simulink model "ship_surface"  (R2026a)
settings: configuration reference "standardSILConfiguraitonParams" (kept outside this file)
undefined symbols (not defined in the file): vehicleParams
settings Model: Creator=jerem  LastModifiedBy=Edison Altamirano
settings ConfigSetRef: SourceName=standardSILConfiguraitonParams  SourceLocation=Base Workspace

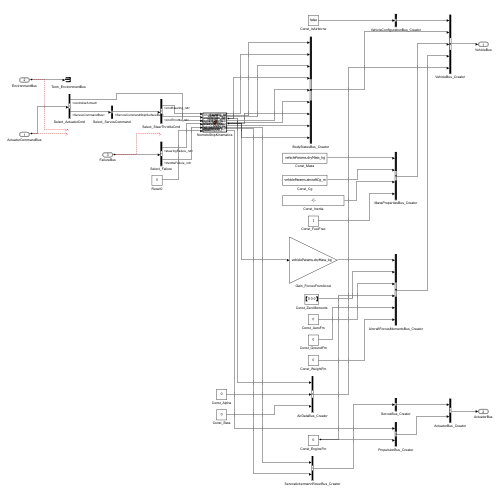
[thumbnail: Simulink's stored preview of the top-level diagram]
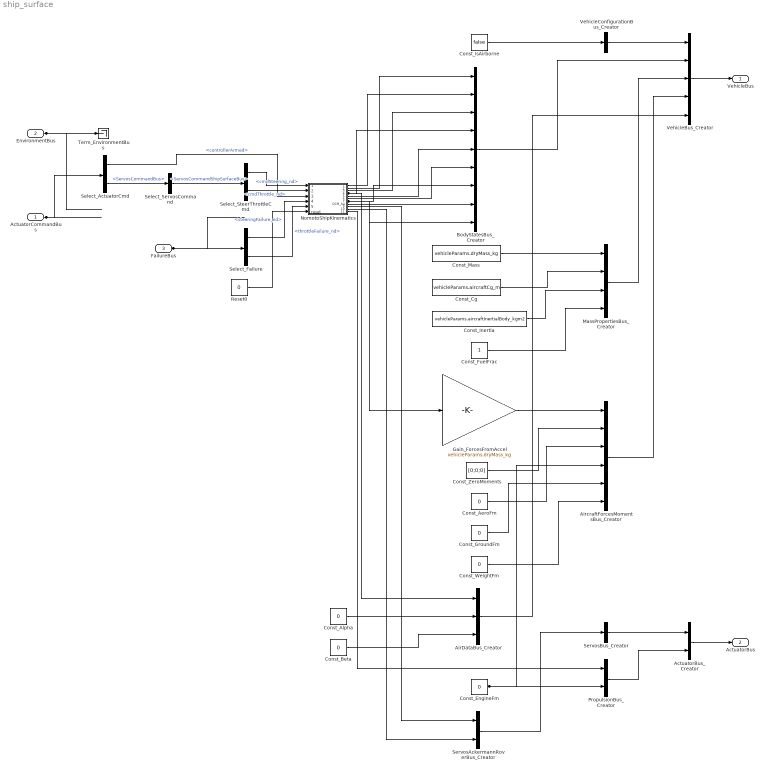
== system ship_surface ==
  ActuatorCommandBus : Inport  OutDataTypeStr=Bus: ActuatorCommandBus
  EnvironmentBus : Inport  Port=2  OutDataTypeStr=Bus: EnvironmentBus
  FailureBus : Inport  Port=3  OutDataTypeStr=Bus: FailureBus
  ActuatorBus_Creator : BusCreator  Inputs=2  OutDataTypeStr=Bus: ActuatorBus
  AirDataBus_Creator : BusCreator  Inputs=3  OutDataTypeStr=Bus: AirDataBus
  AircraftForcesMomentsBus_Creator : BusCreator  Inputs=6  OutDataTypeStr=Bus: AircraftForcesMomentsBus
  BodyStatesBus_Creator : BusCreator  Inputs=9  OutDataTypeStr=Bus: BodyStateBus
  Const_AeroFm : Constant  Value=0  OutDataTypeStr=Bus: ComponentForcesMomentsBus
  Const_Alpha : Constant  Value=0
  Const_Beta : Constant  Value=0
  Const_Cg : Constant  Value=vehicleParams.aircraftCg_m
  Const_EngineFm : Constant  Value=0  OutDataTypeStr=Bus: ComponentForcesMomentsBus
  Const_FuelFrac : Constant
  Const_GroundFm : Constant  Value=0  OutDataTypeStr=Bus: ComponentForcesMomentsBus
  Const_Inertia : Constant  Value=vehicleParams.aircraftInertialBody_kgm2
  Const_IsAirborne : Constant  Value=false  OutDataTypeStr=boolean
  Const_Mass : Constant  Value=vehicleParams.dryMass_kg
  Const_WeightFm : Constant  Value=0  OutDataTypeStr=Bus: ComponentForcesMomentsBus
  Const_ZeroMoments : Constant  Value=[0;0;0]
  Gain_ForcesFromAccel : Gain  Gain=vehicleParams.dryMass_kg
  MassPropertiesBus_Creator : BusCreator  Inputs=4  OutDataTypeStr=Bus: MassPropertiesBus
  NomotoShipKinematics : MATLAB Function  TreatAsAtomicUnit=on
  PropulsionBus_Creator : BusCreator  Inputs=2  OutDataTypeStr=Bus: PropulsionBus
  Reset0 : Constant  Value=0
  Select_ActuatorCmd : BusSelector  OutputSignals=controllerArmed,ServosCommandBus
  Select_Failure : BusSelector  OutputSignals=steeringFailure_nd,throttleFailure_nd
  Select_ServosCommand : BusSelector  OutputSignals=ServosCommandShipSurfaceBus
  Select_SteerThrottleCmd : BusSelector  OutputSignals=cmdSteering_nd,cmdThrottle_nd
  ServosAckermannRoverBus_Creator : BusCreator  Inputs=2  OutDataTypeStr=Bus: ServosShipSurfaceBus
  ServosBus_Creator : BusCreator  Inputs=1  OutDataTypeStr=Bus: ServosBus
  Term_EnvironmentBus : Terminator
  VehicleBus_Creator : BusCreator  Inputs=5  OutDataTypeStr=Bus: VehicleBus
  VehicleConfigurationBus_Creator : BusCreator  Inputs=1  OutDataTypeStr=Bus: VehicleConfigurationBus
  VehicleBus : Outport  OutDataTypeStr=Bus: VehicleBus
  ActuatorBus : Outport  Port=2  OutDataTypeStr=Bus: ActuatorBus
  wires:
  EnvironmentBus/1 -> Term_EnvironmentBus/1
  PropulsionBus_Creator/1 -> ActuatorBus_Creator/2
  NomotoShipKinematics/4(velBody_mps) -> BodyStatesBus_Creator/4, AirDataBus_Creator/1
  ActuatorCommandBus/1 -> Select_ActuatorCmd/1
  Select_ActuatorCmd/1 -> NomotoShipKinematics/3(controllerArmed)  "<controllerArmed>"
  Select_SteerThrottleCmd/2 -> NomotoShipKinematics/2(cmdThrottle_nd)  "<cmdThrottle_nd>"
  Select_SteerThrottleCmd/1 -> NomotoShipKinematics/1(cmdSteering_nd)  "<cmdSteering_nd>"
  Select_Failure/2 -> NomotoShipKinematics/5(throttleFailure_nd)  "<throttleFailure_nd>"
  Select_ServosCommand/1 -> Select_SteerThrottleCmd/1  "<ServosCommandShipSurfaceBus>"
  Const_Cg/1 -> MassPropertiesBus_Creator/2
  Select_ActuatorCmd/2 -> Select_ServosCommand/1  "<ServosCommandBus>"
  FailureBus/1 -> Select_Failure/1
  Select_Failure/1 -> NomotoShipKinematics/4(steeringFailure_nd)  "<steeringFailure_nd>"
  Reset0/1 -> NomotoShipKinematics/6(reset)
  NomotoShipKinematics/5(angVelBody_radps) -> BodyStatesBus_Creator/5
  NomotoShipKinematics/1(posNED_m) -> BodyStatesBus_Creator/2
  NomotoShipKinematics/2(velNED_mps) -> BodyStatesBus_Creator/1
  NomotoShipKinematics/3(eulerAngles_rad) -> BodyStatesBus_Creator/3
  NomotoShipKinematics/6(angAccelBody_radps2) -> BodyStatesBus_Creator/6
  NomotoShipKinematics/7(accelBody_mps2) -> BodyStatesBus_Creator/7, BodyStatesBus_Creator/9, Gain_ForcesFromAccel/1
  NomotoShipKinematics/8(DCM_be) -> BodyStatesBus_Creator/8
  NomotoShipKinematics/9(steeringAngle_rad) -> ServosAckermannRoverBus_Creator/1
  Const_IsAirborne/1 -> VehicleConfigurationBus_Creator/1
  NomotoShipKinematics/10(wheelSpeed_radps) -> ServosAckermannRoverBus_Creator/2
  NomotoShipKinematics/11(motorAngVel_radps) -> PropulsionBus_Creator/1
  Const_WeightFm/1 -> AircraftForcesMomentsBus_Creator/6
  Const_Alpha/1 -> AirDataBus_Creator/2
  Const_Beta/1 -> AirDataBus_Creator/3
  BodyStatesBus_Creator/1 -> VehicleBus_Creator/2
  Const_Mass/1 -> MassPropertiesBus_Creator/1
  Const_GroundFm/1 -> AircraftForcesMomentsBus_Creator/5
  Const_ZeroMoments/1 -> AircraftForcesMomentsBus_Creator/2
  Const_Inertia/1 -> MassPropertiesBus_Creator/3
  Const_FuelFrac/1 -> MassPropertiesBus_Creator/4
  Gain_ForcesFromAccel/1 -> AircraftForcesMomentsBus_Creator/1
  Const_AeroFm/1 -> AircraftForcesMomentsBus_Creator/3
  AirDataBus_Creator/1 -> VehicleBus_Creator/5
  Const_EngineFm/1 -> AircraftForcesMomentsBus_Creator/4, PropulsionBus_Creator/2
  ServosAckermannRoverBus_Creator/1 -> ServosBus_Creator/1
  VehicleConfigurationBus_Creator/1 -> VehicleBus_Creator/1
  MassPropertiesBus_Creator/1 -> VehicleBus_Creator/3
  AircraftForcesMomentsBus_Creator/1 -> VehicleBus_Creator/4
  ServosBus_Creator/1 -> ActuatorBus_Creator/1
  VehicleBus_Creator/1 -> VehicleBus/1
  ActuatorBus_Creator/1 -> ActuatorBus/1

== matlab function ship_surface/NomotoShipKinematics ==
  data: cmdSteering_nd input; posNED_m output; cmdThrottle_nd input; controllerArmed input; steeringFailure_nd input; throttleFailure_nd input; reset input; velNED_mps output; eulerAngles_rad output; velBody_mps output; angVelBody_radps output; angAccelBody_radps2 output; accelBody_mps2 output; DCM_be output; steeringAngle_rad output; wheelSpeed_radps output; motorAngVel_radps output
function [posNED_m, velNED_mps, eulerAngles_rad, velBody_mps, angVelBody_radps, angAccelBody_radps2, accelBody_mps2, DCM_be, steeringAngle_rad, wheelSpeed_radps, motorAngVel_radps] = NomotoShipKinematics(cmdSteering_nd, cmdThrottle_nd, controllerArmed, steeringFailure_nd, throttleFailure_nd, reset)
%#codegen
persistent posN posE yaw speed rudderAng yawRate
if isempty(posN) || reset
    posN = 0; posE = 0; yaw = 1.9199; speed = 0; rudderAng = 0; yawRate = 0;
end
Ts = 0.004;
maxRudderAngle_rad = 0.61;
maxSpeed_mps = 8.0;
tauRudder_s = 3.0;
tauThrottle_s = 30.0;
nomotoK = 0.0229;
nomotoT = 43.75;
propellerGearRatio = 10.0;
referenceAltitude_m = 0;
if steeringFailure_nd
    rudderCmd_rad = rudderAng;
else
    rudderCmd_rad = cmdSteering_nd * maxRudderAngle_rad;
end
if throttleFailure_nd || ~controllerArmed
    speedCmd_mps = 0;
else
    speedCmd_mps = cmdThrottle_nd * maxSpeed_mps;
end
speedDot = (speedCmd_mps - speed) / tauThrottle_s;
yawRateDot = (nomotoK * rudderAng - yawRate) / nomotoT;
posN = posN + Ts * speed * cos(yaw);
posE = posE + Ts * speed * sin(yaw);
yaw = yaw + Ts * yawRate;
speed = speed + Ts * speedDot;
rudderAng = rudderAng + Ts * (rudderCmd_rad - rudderAng) / tauRudder_s;
yawRate = yawRate + Ts * yawRateDot;
posNED_m = [posN; posE; -referenceAltitude_m];
velNED_mps = [speed*cos(yaw); speed*sin(yaw); 0];
eulerAngles_rad = [0; 0; yaw];
velBody_mps = [speed; 0; 0];
angVelBody_radps = [0; 0; yawRate];
angAccelBody_radps2 = [0; 0; yawRateDot];
accelBody_mps2 = [speedDot; speed*yawRate; 0];
DCM_be = [cos(yaw) sin(yaw) 0; -sin(yaw) cos(yaw) 0; 0 0 1];
steeringAngle_rad = rudderAng;
wheelSpeed_radps = speed * propellerGearRatio;
motorAngVel_radps = wheelSpeed_radps;
end
